simulink model "NPC_ANPC_Final_C_Thyristors"  (R2022b)
settings: Solver=VariableStepAuto  StartTime=0.0  StopTime=1  FixedStep=1e-6  RelTol=1e-3
InitFcn:
  | v=3000
  | r=0.000001
  | c=1000e-6
  | l=314
  | i=1000
  | r1=1000
  | t=1/3000
  | ma=2
  | f=2*pi*50
  | p1=(2*pi)/3
  | p2=-(2*pi)/3
libraries: simulink x18, spsIGBTDiodeLib x13, spsRMSLib x9, spsSeriesRLCBranchLib x9, spsTHDLib x9, spsDiodeLib x6, spsMeanLib x3, spsVoltageMeasurementLib x3, spsCurrentMeasurementLib x2, spsThreePhaseVIMeasurementLib x2, spsUniversalBridgeLib x2, spspowerguiLib x2
settings Model: Creator=dell  LastModifiedBy=shubh
settings SolverCC: ZeroCrossAlgorithm=Adaptive  AlgebraicLoopSolver=TrustRegion
settings DataIOCC: ReturnWorkspaceOutputs=off
settings DebuggingCC: MaskedZcDiagnostic=none  IgnoredZcDiagnostic=none  UnconnectedInputMsg=warning  UnconnectedOutputMsg=warning  UnconnectedLineMsg=warning  SFMachineParentedDataDiag=warning  ArithmeticOperatorsInVariantConditions=warning
settings ModelReferenceCC: EnableRefExpFcnMdlSchedulingChecks=on
settings SFSimCC: SimUseLocalCustomCode=off  CustomCodeUndefinedFunction=UseInterfaceOnly
settings RTWCC: RTWUseLocalCustomCode=off
settings CodeAppCC: StateflowObjectComments=on
settings SimscapeCC: SimscapeNormalizeSystem=off

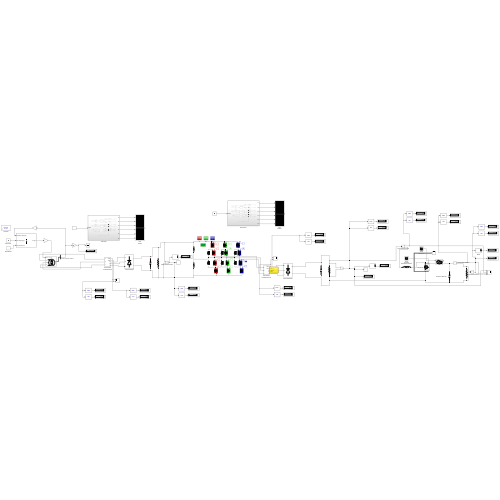
[thumbnail: Simulink's stored preview of the top-level diagram]
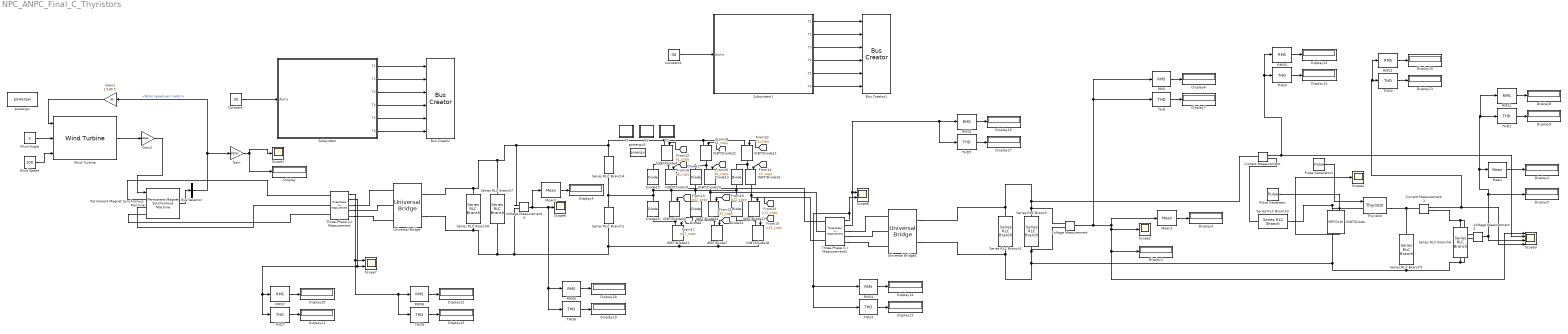
== system NPC_ANPC_Final_C_Thyristors ==
  A2 : Subsystem
  B2 : Subsystem
  Bus Creator : BusCreator  Inputs=6
  Bus Creator1 : BusCreator  Inputs=6
  Bus Selector : BusSelector  OutputSignals=Rotor speed wm (rad/s)
  C2 : Subsystem
  Constant : Constant  Value=-30
  Constant1 : Constant  Value=-30
  Current Measurement : spsCurrentMeasurementLib/Current Measurement  PhasorSimulation=off  OutputType=Complex  PSBequivalent=0
  Current Measurement1 : spsCurrentMeasurementLib/Current Measurement  PhasorSimulation=off  OutputType=Complex  PSBequivalent=0
  Diode{6,13..17} (6 alike) : spsDiodeLib/Diode  Ron=0.001  Lon=0  Vf=0.8  IC=0  UseSnubber=0  Rs=500  Cs=250e-9  Measurements=off
  Display{,1..23} (24 alike) : Display
  Gain : Gain  Gain=30/pi
  Gain1 : Gain  Gain=1/188.5
  Gain2 : Gain  Gain=19643
  IGBT/Diode : spsIGBTDiodeLib/IGBT//Diode  Ron=1e-3  Rs=1e5  Cs=inf  Measurements=on
  IGBT/Diode{4,7,11,16..24} (12 alike) : spsIGBTDiodeLib/IGBT//Diode  Ron=1e-3  Rs=1e5  Cs=inf  Measurements=off
  Mean : spsMeanLib/Mean  Freq=60  Vinit=0  Ts=0
      link override Model/integrator: InitialCondition=0  AbsoluteTolerance=1e-4
  Mean1 : spsMeanLib/Mean  Freq=60  Vinit=0  Ts=0
  Mean2 : spsMeanLib/Mean  Freq=60  Vinit=0  Ts=0
  Permanent Magnet Synchronous Machine : spsPermanentMagnetSynchronousMachineLib/Permanent Magnet Synchronous Machine  NbPhases=3  FluxDistribution=Sinusoidal  RotorType=Round  MechanicalLoad=Torque Tm  PresetModel=No  ShowDetailedParameters=on  MeasurementBus=off  Resistance=0.0485  Inductance=8.5e-3  dqInductances=[8.5e-3,8.5e-3]  La=0.000395  MachineConstant=Flux linkage established by magnets (V.s)  Flux=0.1194  VoltageCst=86.6271  TorqueCst=0.7164  Flat=120  Mechanical=[0.0027 0.0004924 4 0]  PolePairs=4  InitialConditions=[0,0, 0,0]  InitialConditions5ph=[0 0 0 0 0 0]  RefAngle=90 degrees behind phase A axis (modified Park)  IterativeDiscreteModel=Trapezoidal non iterative  TsBlock=-1  TsPowergui=0
  Pitch Angle : Constant  Value=3
  Pulse Generator : DiscretePulseGenerator  PulseType=Time based  Amplitude=4  Period=1/5000  PulseWidth=60
  Pulse Generator1 : DiscretePulseGenerator  PulseType=Time based  Amplitude=4  Period=1/5000  PulseWidth=60  PhaseDelay=45*(1/5000)/180
  RMS{,1..8} (9 alike) : spsRMSLib/RMS  TrueRMS=on  Freq=60  RMSInit=120  Ts=0
  Scope{1..2,4,6} (4 alike) : Scope
  Scope3 : Scope  NumInputPorts=4
  Scope7 : Scope  NumInputPorts=2
  Scope8 : Scope  NumInputPorts=2
  Series RLC Branch : spsSeriesRLCBranchLib/Series RLC Branch  LConnTagsString=__new0  RConnTagsString=__new0  BranchType=R  Resistance=10  Inductance=1e-3  SetiL0=off  InitialCurrent=0  Capacitance=1e-6  Setx0=off  InitialVoltage=0  Measurements=None
  Series RLC Branch1 : spsSeriesRLCBranchLib/Series RLC Branch  LConnTagsString=__new0  RConnTagsString=__new0  BranchType=C  Resistance=10  Inductance=10e-3  SetiL0=off  InitialCurrent=0  Capacitance=10e-3  Setx0=off  InitialVoltage=0  Measurements=None
  Series RLC Branch2 : spsSeriesRLCBranchLib/Series RLC Branch  LConnTagsString=__new0  RConnTagsString=__new0  BranchType=C  Resistance=1  Inductance=1e-3  SetiL0=off  InitialCurrent=0  Capacitance=10e-9  Setx0=off  InitialVoltage=i  Measurements=None
  Series RLC Branch3 : spsSeriesRLCBranchLib/Series RLC Branch  LConnTagsString=__new0  RConnTagsString=__new0  BranchType=L  Resistance=1  Inductance=6e-3  SetiL0=off  InitialCurrent=0  Capacitance=1e-6  Setx0=off  InitialVoltage=0  Measurements=None
  Series RLC Branch4 : spsSeriesRLCBranchLib/Series RLC Branch  LConnTagsString=__new0  RConnTagsString=__new0  BranchType=C  Resistance=1  Inductance=1e-3  SetiL0=off  InitialCurrent=0  Capacitance=10e-9  Setx0=off  InitialVoltage=i  Measurements=None
  Series RLC Branch5 : spsSeriesRLCBranchLib/Series RLC Branch  LConnTagsString=__new0  RConnTagsString=__new0  BranchType=C  Resistance=1  Inductance=6e-3  SetiL0=off  InitialCurrent=0  Capacitance=5000e-6  Setx0=off  InitialVoltage=0  Measurements=None
  Series RLC Branch6 : spsSeriesRLCBranchLib/Series RLC Branch  LConnTagsString=__new0  RConnTagsString=__new0  BranchType=R  Resistance=12.5  Inductance=6e-08  SetiL0=off  InitialCurrent=0  Capacitance=1e-6  Setx0=off  InitialVoltage=0  Measurements=None
  Series RLC Branch7 : spsSeriesRLCBranchLib/Series RLC Branch  LConnTagsString=__new0  RConnTagsString=__new0  BranchType=R  Resistance=10  Inductance=10e-3  SetiL0=off  InitialCurrent=0  Capacitance=10e-3  Setx0=off  InitialVoltage=0  Measurements=None
  Series RLC Branch8 : spsSeriesRLCBranchLib/Series RLC Branch  LConnTagsString=__new0  RConnTagsString=__new0  BranchType=C  Resistance=10  Inductance=10e-3  SetiL0=off  InitialCurrent=0  Capacitance=10e-3  Setx0=off  InitialVoltage=0  Measurements=None
  Subsystem : Subsystem
  Subsystem1 : Subsystem
  THD{,1..8} (9 alike) : spsTHDLib/THD  Freq=60  Ts=0
  Three-Phase V-I Measurement : spsThreePhaseVIMeasurementLib/Three-Phase V-I Measurement  VoltageMeasurement=phase-to-phase  SetLabelV=off  LabelV=Vabc  Vpu=off  VpuLL=off  CurrentMeasurement=yes  SetLabelI=off  LabelI=Iabc  Ipu=off  Pbase=100e6  Vbase=500e3  OutputType=Complex  PhasorSimulation=off  PSBequivalent=0
  Three-Phase V-I Measurement2 : spsThreePhaseVIMeasurementLib/Three-Phase V-I Measurement  VoltageMeasurement=phase-to-phase  SetLabelV=off  LabelV=Vabc  Vpu=off  VpuLL=off  CurrentMeasurement=yes  SetLabelI=off  LabelI=Iabc  Ipu=off  Pbase=100e6  Vbase=500e3  OutputType=Complex  PhasorSimulation=off  PSBequivalent=0
  Thyristor : spsThyristorLib/Thyristor  Ron=0.001  Lon=0  Vf=0.8  IC=0  Rs=500  Cs=250e-9  Measurements=on
  Universal Bridge : spsUniversalBridgeLib/Universal Bridge  Arms=3  SnubberResistance=1e5  SnubberCapacitance=inf  Device=Diodes  Ron=1e-3  Lon=0  ForwardVoltages="[  0  0  ]"  ForwardVoltage=0  GTOparameters=[ 10e-6 , 20e-6 ]  IGBTparameters=[ 1e-6 , 2e-6 ]  Measurements=None  Measurements_2=None  converterType=Rectifier
  Universal Bridge1 : spsUniversalBridgeLib/Universal Bridge  Arms=3  SnubberResistance=1e5  SnubberCapacitance=inf  Device=Diodes  Ron=1e-3  Lon=0  ForwardVoltages="[  0  0  ]"  ForwardVoltage=0  GTOparameters=[ 10e-6 , 20e-6 ]  IGBTparameters=[ 1e-6 , 2e-6 ]  Measurements=None  Measurements_2=None  converterType=Rectifier
  Voltage Measurement : spsVoltageMeasurementLib/Voltage Measurement  PhasorSimulation=off  OutputType=Complex  PSBequivalent=0
  Voltage Measurement2 : spsVoltageMeasurementLib/Voltage Measurement  PhasorSimulation=off  OutputType=Complex  PSBequivalent=0
  Voltage Measurement3 : spsVoltageMeasurementLib/Voltage Measurement  PhasorSimulation=off  OutputType=Complex  PSBequivalent=0
  Wind Speed : Constant  Value=100
  Wind Turbine : spsWindTurbineLib/Wind Turbine  Pnom=1.5e6  Pelec_base=1.5e6/0.9  wind_base=12  P_wind_base=0.73  speed_nom=1.2  pitch_angle=0  c1_c6="[0.51763          116          0.4            5           21     0.006795]"  cp_nom=0.48  lambda_nom=8.1
  powergui : spspowerguiLib/powergui  Priority=1  SimulationMode=Discrete  SampleTime=1e-6  frequency=60  Iterations=50  frequencyindice=0  Pbase=100e6  ErrMax=1e-4  UnitsV=kV  UnitsW=MW  buscounter=0  FunctionMessages=off  echomessages=off  EnableUseOfTLC=off  CurrentSourceSwitches=off  DisableSnubberDevices=off  DisableRonSwitches=off  DisableVfSwitches=off  DisplayEquations=off  AutomaticDiscreteSolvers=off  SolverType=Tustin/Backward Euler (TBE)  Interpol=off  ExternalGateDelay=off  methode=off  Ts=100  x0status=blocks  SPID=on  SwTol=0  HookPort=off  NonlinearTolerance=1e-4  nMaxIteration=100  ContinueOnMaxIteration=off  RestoreLinks=warning  ResistiveCurrentMeasurement=off  Frange=[0:2:500]  Ylog=off  Xlog=on  ShowGrid=off  save=off  variable=ZData  structure=0  ZoomFFT=off  StartTime=0.0  cycles=1  DisplayStyle=1  fundamental=60  FreqAxis=off  MaxFrequency=1000  frequencyindicesteady=1  RmsSteady=1  display=off
  powergui1 : spspowerguiLib/powergui  Priority=1  SimulationMode=Discrete  SampleTime=1e-6  frequency=60  Iterations=50  frequencyindice=0  Pbase=100e6  ErrMax=1e-4  UnitsV=kV  UnitsW=MW  buscounter=0  FunctionMessages=off  echomessages=off  EnableUseOfTLC=off  CurrentSourceSwitches=off  DisableSnubberDevices=off  DisableRonSwitches=off  DisableVfSwitches=off  DisplayEquations=off  AutomaticDiscreteSolvers=off  SolverType=Tustin/Backward Euler (TBE)  Interpol=off  ExternalGateDelay=off  methode=off  Ts=100  x0status=blocks  SPID=on  SwTol=0  HookPort=off  NonlinearTolerance=1e-4  nMaxIteration=100  ContinueOnMaxIteration=off  RestoreLinks=warning  ResistiveCurrentMeasurement=off  Frange=[0:2:500]  Ylog=off  Xlog=on  ShowGrid=off  save=off  variable=ZData  structure=d  ZoomFFT=off  StartTime=0.2  cycles=2  DisplayStyle=1  fundamental=50  FreqAxis=on  MaxFrequency=40000  frequencyindicesteady=1  RmsSteady=1  display=off
  wires:
  Mean1/1 -> Display3/1
  Mean2/1 -> Display4/1
  [a2_copy] -> IGBT/Diode19/1
  Current Measurement/1 -> THD3/1, RMS3/1, Scope3/2
  [c2_copy] -> IGBT/Diode16/1
  Current Measurement1/1 -> RMS2/1, THD2/1, Scope3/4
  Subsystem/5(T5) -> Bus Creator/5
  Subsystem/6(T6) -> Bus Creator/6
  IGBT/Diode/1 -> Scope4/1
  Subsystem/3(T3) -> Bus Creator/3
  Constant/1 -> Subsystem/1(Alpha)
  Subsystem/2(T2) -> Bus Creator/2
  Subsystem/4(T4) -> Bus Creator/4
  [a1_copy] -> IGBT/Diode4/1
  [b1_copy] -> IGBT/Diode22/1
  Three-Phase V-I Measurement/1 -> THD8/1, RMS8/1, Scope7/1
  Subsystem1/5(T5) -> Bus Creator1/5
  Subsystem1/4(T4) -> Bus Creator1/4
  Mean/1 -> Display2/1
  [c22_copy] -> IGBT/Diode18/1
  [b22_copy] -> IGBT/Diode7/1
  Subsystem1/3(T3) -> Bus Creator1/3
  Three-Phase V-I Measurement/2 -> Scope7/2, THD7/1, RMS7/1
  Subsystem1/6(T6) -> Bus Creator1/6
  Subsystem1/2(T2) -> Bus Creator1/2
  Subsystem1/1(T1) -> Bus Creator1/1
  Pulse Generator/1 -> IGBT/Diode/1
  [a11_copy] -> IGBT/Diode20/1
  [a22_copy] -> IGBT/Diode21/1
  Voltage Measurement/1 -> RMS/1, THD/1, Scope3/1, Display1/1, Scope2/1, Mean1/1
  Constant1/1 -> Subsystem1/1(Alpha)
  [b11_copy] -> IGBT/Diode24/1
  Subsystem/1(T1) -> Bus Creator/1
  Voltage Measurement3/1 -> THD6/1, RMS6/1, Scope6/1, Mean2/1
  [b2_copy] -> IGBT/Diode23/1
  [c1_copy] -> IGBT/Diode11/1
  [c11_copy] -> IGBT/Diode17/1
  Pitch Angle/1 -> Wind Turbine/2
  Bus Selector/1 -> Gain1/1, Gain/1  "<Rotor speed wm (rad/s)>"
  Permanent Magnet Synchronous Machine/1 -> Bus Selector/1
  Gain/1 -> Display/1, Scope1/1
  Wind Speed/1 -> Wind Turbine/3
  Three-Phase V-I Measurement2/2 -> THD5/1, RMS5/1, Scope8/1
  Pulse Generator1/1 -> Thyristor/1
  Voltage Measurement2/1 -> Display5/1, RMS1/1, THD1/1, Mean/1, Scope3/3
  Gain1/1 -> Wind Turbine/1
  Wind Turbine/1 -> Gain2/1
  Gain2/1 -> Permanent Magnet Synchronous Machine/1
  RMS/1 -> Display6/1
  THD/1 -> Display7/1
  RMS1/1 -> Display8/1
  THD1/1 -> Display9/1
  RMS2/1 -> Display10/1
  THD2/1 -> Display11/1
  RMS3/1 -> Display12/1
  THD3/1 -> Display13/1
  RMS4/1 -> Display14/1
  THD4/1 -> Display15/1
  Three-Phase V-I Measurement2/1 -> THD4/1, RMS4/1, Scope8/2
  RMS5/1 -> Display16/1
  THD5/1 -> Display17/1
  RMS6/1 -> Display18/1
  THD6/1 -> Display19/1
  RMS7/1 -> Display20/1
  THD7/1 -> Display21/1
  RMS8/1 -> Display22/1
  THD8/1 -> Display23/1
  connections:
  Diode6/LConn1 -- IGBT/Diode24/RConn1 -- IGBT/Diode7/LConn1
  Voltage Measurement2/LConn1 -- Current Measurement1/RConn1 -- Series RLC Branch6/LConn1
  IGBT/Diode21/RConn1 -- IGBT/Diode18/RConn1 -- IGBT/Diode7/RConn1 -- Series RLC Branch8/RConn1 -- Universal Bridge/RConn2 -- Series RLC Branch7/RConn1 -- Voltage Measurement3/LConn2 -- Series RLC Branch2/LConn1
  Series RLC Branch3/LConn1 -- IGBT/Diode/LConn1 -- Thyristor/LConn1
  Series RLC Branch2/RConn1 -- Series RLC Branch4/LConn1 -- Diode16/RConn1 -- Diode13/LConn1 -- Diode14/RConn1 -- Diode6/RConn1 -- Diode17/LConn1 -- Diode15/LConn1
  Diode13/RConn1 -- IGBT/Diode11/RConn1 -- IGBT/Diode16/LConn1
  Diode15/RConn1 -- IGBT/Diode4/RConn1 -- IGBT/Diode19/LConn1
  Series RLC Branch8/LConn1 -- Universal Bridge/RConn1 -- Series RLC Branch7/LConn1 -- Voltage Measurement3/LConn1 -- Series RLC Branch4/RConn1 -- IGBT/Diode4/LConn1 -- IGBT/Diode11/LConn1 -- IGBT/Diode22/LConn1
  Three-Phase V-I Measurement2/LConn2 -- IGBT/Diode24/LConn1 -- IGBT/Diode23/RConn1
  Current Measurement1/LConn1 -- Thyristor/RConn1 -- Series RLC Branch5/LConn1
  Universal Bridge1/RConn1 -- Series RLC Branch1/LConn1 -- Voltage Measurement/LConn1 -- Series RLC Branch/LConn1 -- Current Measurement/LConn1
  Series RLC Branch6/RConn1 -- IGBT/Diode/RConn1 -- Universal Bridge1/RConn2 -- Series RLC Branch1/RConn1 -- Voltage Measurement/LConn2 -- Series RLC Branch/RConn1 -- Series RLC Branch5/RConn1 -- Voltage Measurement2/LConn2
  Three-Phase V-I Measurement2/LConn1 -- IGBT/Diode20/LConn1 -- IGBT/Diode19/RConn1
  Diode16/LConn1 -- IGBT/Diode20/RConn1 -- IGBT/Diode21/LConn1
  Diode17/RConn1 -- IGBT/Diode22/RConn1 -- IGBT/Diode23/LConn1
  IGBT/Diode17/LConn1 -- IGBT/Diode16/RConn1 -- Three-Phase V-I Measurement2/LConn3
  Diode14/LConn1 -- IGBT/Diode17/RConn1 -- IGBT/Diode18/LConn1
  Three-Phase V-I Measurement/RConn2 -- Universal Bridge/LConn2
  Series RLC Branch3/RConn1 -- Current Measurement/RConn1
  Three-Phase V-I Measurement/RConn3 -- Universal Bridge/LConn3
  Three-Phase V-I Measurement/RConn1 -- Universal Bridge/LConn1
  Three-Phase V-I Measurement2/RConn1 -- Universal Bridge1/LConn1
  Three-Phase V-I Measurement2/RConn3 -- Universal Bridge1/LConn3
  Three-Phase V-I Measurement2/RConn2 -- Universal Bridge1/LConn2
  Permanent Magnet Synchronous Machine/LConn1 -- Three-Phase V-I Measurement/LConn1
  Permanent Magnet Synchronous Machine/LConn2 -- Three-Phase V-I Measurement/LConn2
  Permanent Magnet Synchronous Machine/LConn3 -- Three-Phase V-I Measurement/LConn3

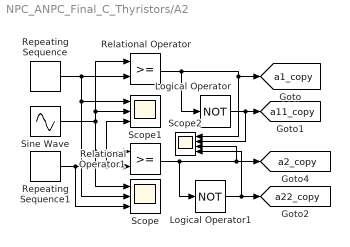
== system NPC_ANPC_Final_C_Thyristors/A2 ==
  Logical Operator : Logic  Operator=NOT  AllPortsSameDT=off  OutDataTypeStr=boolean
  Logical Operator1 : Logic  Operator=NOT  AllPortsSameDT=off  OutDataTypeStr=boolean
  Relational Operator : RelationalOperator  OutDataTypeStr=boolean  RndMeth=Simplest  InputSameDT=off
  Relational Operator1 : RelationalOperator  OutDataTypeStr=boolean  RndMeth=Simplest  InputSameDT=off
  Repeating Sequence : simulink/Sources/Repeating Sequence  rep_seq_t=[0 t/2 t]  rep_seq_y=[0 2 0]
  Repeating Sequence1 : simulink/Sources/Repeating Sequence  rep_seq_t=[0 t/2 t]  rep_seq_y=[-2 0 -2]
  Scope : Scope  NumInputPorts=3
  Scope1 : Scope  NumInputPorts=3
  Scope2 : Scope  NumInputPorts=4
  Sine Wave : Sin  Amplitude=ma  Frequency=f  SampleTime=0
  tag scope: a11_copy=global, a1_copy=global, a22_copy=global, a2_copy=global
  wires:
  Sine Wave/1 -> Relational Operator/1, Scope1/2, Relational Operator1/1, Scope/1
  Relational Operator1/1 -> [a2_copy], Scope2/3, Logical Operator1/1
  Relational Operator/1 -> Logical Operator/1, [a1_copy], Scope2/1
  Repeating Sequence1/1 -> Relational Operator1/2, Scope1/3, Scope/3
  Repeating Sequence/1 -> Relational Operator/2, Scope/2, Scope1/1
  Logical Operator1/1 -> Scope2/4, [a22_copy]
  Logical Operator/1 -> [a11_copy], Scope2/2

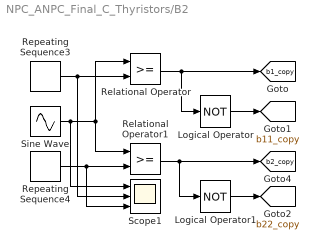
== system NPC_ANPC_Final_C_Thyristors/B2 ==
  Logical Operator : Logic  Operator=NOT  AllPortsSameDT=off  OutDataTypeStr=boolean
  Logical Operator1 : Logic  Operator=NOT  AllPortsSameDT=off  OutDataTypeStr=boolean
  Relational Operator : RelationalOperator  OutDataTypeStr=boolean  RndMeth=Simplest  InputSameDT=off
  Relational Operator1 : RelationalOperator  OutDataTypeStr=boolean  RndMeth=Simplest  InputSameDT=off
  Repeating Sequence3 : simulink/Sources/Repeating Sequence  rep_seq_t=[0 t/2 t]  rep_seq_y=[0 2 0]
  Repeating Sequence4 : simulink/Sources/Repeating Sequence  rep_seq_t=[0 t/2 t]  rep_seq_y=[-2 0 -2]
  Scope1 : Scope  NumInputPorts=3
  Sine Wave : Sin  Amplitude=ma  Frequency=f  Phase=p2  SampleTime=0
  tag scope: b11_copy=global, b1_copy=global, b22_copy=global, b2_copy=global
  wires:
  Logical Operator/1 -> [b11_copy]
  Relational Operator/1 -> [b1_copy], Logical Operator/1
  Relational Operator1/1 -> [b2_copy], Logical Operator1/1
  Sine Wave/1 -> Relational Operator/1, Relational Operator1/1, Scope1/1
  Repeating Sequence4/1 -> Relational Operator1/2, Scope1/3
  Repeating Sequence3/1 -> Relational Operator/2, Scope1/2
  Logical Operator1/1 -> [b22_copy]

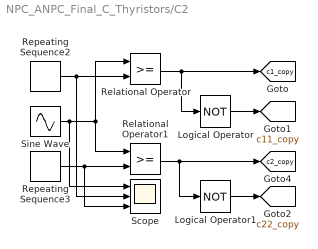
== system NPC_ANPC_Final_C_Thyristors/C2 ==
  Logical Operator : Logic  Operator=NOT  AllPortsSameDT=off  OutDataTypeStr=boolean
  Logical Operator1 : Logic  Operator=NOT  AllPortsSameDT=off  OutDataTypeStr=boolean
  Relational Operator : RelationalOperator  OutDataTypeStr=boolean  RndMeth=Simplest  InputSameDT=off
  Relational Operator1 : RelationalOperator  OutDataTypeStr=boolean  RndMeth=Simplest  InputSameDT=off
  Repeating Sequence2 : simulink/Sources/Repeating Sequence  rep_seq_t=[0 t/2 t]  rep_seq_y=[0 2 0]
  Repeating Sequence3 : simulink/Sources/Repeating Sequence  rep_seq_t=[0 t/2 t]  rep_seq_y=[-2 0 -2]
  Scope : Scope  NumInputPorts=3
  Sine Wave : Sin  Amplitude=ma  Frequency=f  Phase=p1  SampleTime=0
  tag scope: c11_copy=global, c1_copy=global, c22_copy=global, c2_copy=global
  wires:
  Logical Operator/1 -> [c11_copy]
  Relational Operator/1 -> [c1_copy], Logical Operator/1
  Relational Operator1/1 -> [c2_copy], Logical Operator1/1
  Sine Wave/1 -> Relational Operator/1, Relational Operator1/1, Scope/1
  Repeating Sequence3/1 -> Relational Operator1/2, Scope/3
  Repeating Sequence2/1 -> Relational Operator/2, Scope/2
  Logical Operator1/1 -> [c22_copy]

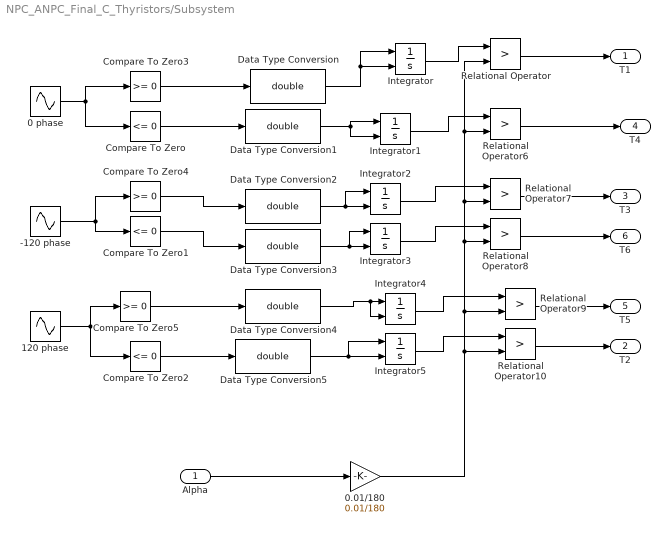
== system NPC_ANPC_Final_C_Thyristors/Subsystem ==
  Alpha : Inport
  -120 phase : Sin  Frequency=100*pi  Phase=-120*(pi/180)  SampleTime=0
  0 phase : Sin  Frequency=100*pi  SampleTime=0
  0.01/180 : Gain  Gain=0.01/180
  120 phase : Sin  Frequency=100*pi  Phase=+120*(pi/180)  SampleTime=0
  Compare To Zero : simulink/Logic and Bit Operations/Compare To Zero  relop=<=  OutDataTypeStr=boolean
  Compare To Zero1 : simulink/Logic and Bit Operations/Compare To Zero  relop=<=  OutDataTypeStr=boolean
  Compare To Zero2 : simulink/Logic and Bit Operations/Compare To Zero  relop=<=  OutDataTypeStr=boolean
  Compare To Zero3 : simulink/Logic and Bit Operations/Compare To Zero  relop=>=  OutDataTypeStr=boolean
  Compare To Zero4 : simulink/Logic and Bit Operations/Compare To Zero  relop=>=  OutDataTypeStr=boolean
  Compare To Zero5 : simulink/Logic and Bit Operations/Compare To Zero  relop=>=  OutDataTypeStr=boolean
  Data Type Conversion{,1..5} (6 alike) : DataTypeConversion  OutDataTypeStr=double  SaturateOnIntegerOverflow=off  RndMeth=Floor
  Integrator{,1..5} (6 alike) : Integrator  ExternalReset=falling
  Relational Operator{,6..10} (6 alike) : RelationalOperator  Operator=>  OutDataTypeStr=boolean  RndMeth=Simplest  InputSameDT=off
  T1 : Outport  VectorParamsAs1DForOutWhenUnconnected=off
  T2 : Outport  Port=2  VectorParamsAs1DForOutWhenUnconnected=off
  T3 : Outport  Port=3  VectorParamsAs1DForOutWhenUnconnected=off
  T4 : Outport  Port=4  VectorParamsAs1DForOutWhenUnconnected=off
  T5 : Outport  Port=5  VectorParamsAs1DForOutWhenUnconnected=off
  T6 : Outport  Port=6  VectorParamsAs1DForOutWhenUnconnected=off
  wires:
  Integrator2/1 -> Relational Operator7/1
  0 phase/1 -> Compare To Zero/1, Compare To Zero3/1
  Compare To Zero1/1 -> Data Type Conversion3/1
  Data Type Conversion4/1 -> Integrator4/2, Integrator4/1
  Integrator4/1 -> Relational Operator9/1
  Compare To Zero4/1 -> Data Type Conversion2/1
  Relational Operator9/1 -> T5/1
  Integrator3/1 -> Relational Operator8/1
  Alpha/1 -> 0.01/180/1
  120 phase/1 -> Compare To Zero2/1, Compare To Zero5/1
  Relational Operator10/1 -> T2/1
  Compare To Zero3/1 -> Data Type Conversion/1
  0.01/180/1 -> Relational Operator9/2, Relational Operator8/2, Relational Operator7/2, Relational Operator6/2, Relational Operator/2, Relational Operator10/2
  Data Type Conversion3/1 -> Integrator3/1, Integrator3/2
  Integrator5/1 -> Relational Operator10/1
  -120 phase/1 -> Compare To Zero1/1, Compare To Zero4/1
  Integrator/1 -> Relational Operator/1
  Data Type Conversion2/1 -> Integrator2/2, Integrator2/1
  Data Type Conversion1/1 -> Integrator1/2, Integrator1/1
  Relational Operator/1 -> T1/1
  Data Type Conversion/1 -> Integrator/2, Integrator/1
  Integrator1/1 -> Relational Operator6/1
  Data Type Conversion5/1 -> Integrator5/2, Integrator5/1
  Compare To Zero/1 -> Data Type Conversion1/1
  Relational Operator6/1 -> T4/1
  Compare To Zero5/1 -> Data Type Conversion4/1
  Relational Operator7/1 -> T3/1
  Relational Operator8/1 -> T6/1
  Compare To Zero2/1 -> Data Type Conversion5/1

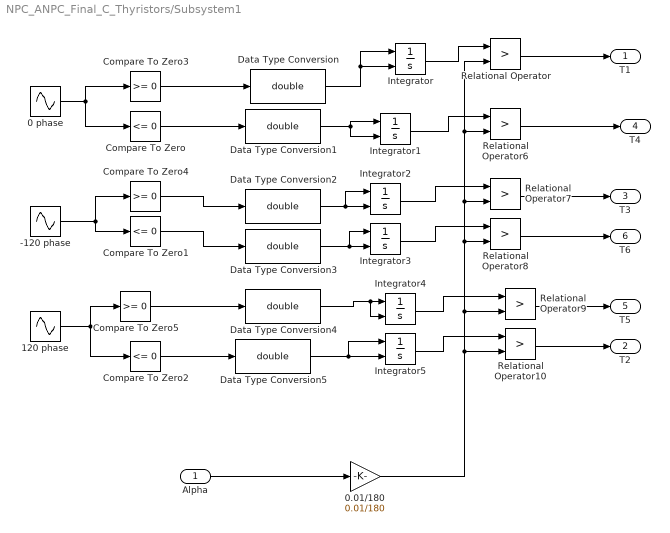
== system NPC_ANPC_Final_C_Thyristors/Subsystem1 ==
  Alpha : Inport
  -120 phase : Sin  Frequency=100*pi  Phase=-120*(pi/180)  SampleTime=0
  0 phase : Sin  Frequency=100*pi  SampleTime=0
  0.01/180 : Gain  Gain=0.01/180
  120 phase : Sin  Frequency=100*pi  Phase=+120*(pi/180)  SampleTime=0
  Compare To Zero : simulink/Logic and Bit Operations/Compare To Zero  relop=<=  OutDataTypeStr=boolean
  Compare To Zero1 : simulink/Logic and Bit Operations/Compare To Zero  relop=<=  OutDataTypeStr=boolean
  Compare To Zero2 : simulink/Logic and Bit Operations/Compare To Zero  relop=<=  OutDataTypeStr=boolean
  Compare To Zero3 : simulink/Logic and Bit Operations/Compare To Zero  relop=>=  OutDataTypeStr=boolean
  Compare To Zero4 : simulink/Logic and Bit Operations/Compare To Zero  relop=>=  OutDataTypeStr=boolean
  Compare To Zero5 : simulink/Logic and Bit Operations/Compare To Zero  relop=>=  OutDataTypeStr=boolean
  Data Type Conversion{,1..5} (6 alike) : DataTypeConversion  OutDataTypeStr=double  SaturateOnIntegerOverflow=off  RndMeth=Floor
  Integrator{,1..5} (6 alike) : Integrator  ExternalReset=falling
  Relational Operator{,6..10} (6 alike) : RelationalOperator  Operator=>  OutDataTypeStr=boolean  RndMeth=Simplest  InputSameDT=off
  T1 : Outport  VectorParamsAs1DForOutWhenUnconnected=off
  T2 : Outport  Port=2  VectorParamsAs1DForOutWhenUnconnected=off
  T3 : Outport  Port=3  VectorParamsAs1DForOutWhenUnconnected=off
  T4 : Outport  Port=4  VectorParamsAs1DForOutWhenUnconnected=off
  T5 : Outport  Port=5  VectorParamsAs1DForOutWhenUnconnected=off
  T6 : Outport  Port=6  VectorParamsAs1DForOutWhenUnconnected=off
  wires:
  Integrator2/1 -> Relational Operator7/1
  0 phase/1 -> Compare To Zero/1, Compare To Zero3/1
  Compare To Zero1/1 -> Data Type Conversion3/1
  Data Type Conversion4/1 -> Integrator4/2, Integrator4/1
  Integrator4/1 -> Relational Operator9/1
  Compare To Zero4/1 -> Data Type Conversion2/1
  Relational Operator9/1 -> T5/1
  Integrator3/1 -> Relational Operator8/1
  Alpha/1 -> 0.01/180/1
  120 phase/1 -> Compare To Zero2/1, Compare To Zero5/1
  Relational Operator10/1 -> T2/1
  Compare To Zero3/1 -> Data Type Conversion/1
  0.01/180/1 -> Relational Operator9/2, Relational Operator8/2, Relational Operator7/2, Relational Operator6/2, Relational Operator/2, Relational Operator10/2
  Data Type Conversion3/1 -> Integrator3/1, Integrator3/2
  Integrator5/1 -> Relational Operator10/1
  -120 phase/1 -> Compare To Zero1/1, Compare To Zero4/1
  Integrator/1 -> Relational Operator/1
  Data Type Conversion2/1 -> Integrator2/2, Integrator2/1
  Data Type Conversion1/1 -> Integrator1/2, Integrator1/1
  Relational Operator/1 -> T1/1
  Data Type Conversion/1 -> Integrator/2, Integrator/1
  Integrator1/1 -> Relational Operator6/1
  Data Type Conversion5/1 -> Integrator5/2, Integrator5/1
  Compare To Zero/1 -> Data Type Conversion1/1
  Relational Operator6/1 -> T4/1
  Compare To Zero5/1 -> Data Type Conversion4/1
  Relational Operator7/1 -> T3/1
  Relational Operator8/1 -> T6/1
  Compare To Zero2/1 -> Data Type Conversion5/1
